simulink library "ox_lib"  (Simulink 7.5)
settings: Solver=ode45  SolverMode=SingleTasking  StartTime=0.0  StopTime=10.0  RelTol=1e-3
PostLoadFcn:
  | % Stub definitions for mask variables
  | delay_depth=16;
  | n_bits=8;
  | bin_pt=7;
libraries: xbsIndex_r4 x698, casper_library x173, ox_lib x8, xps_library x2
(part 1 of 8)
settings Model: Creator=mwagner  LastModifiedBy=jack

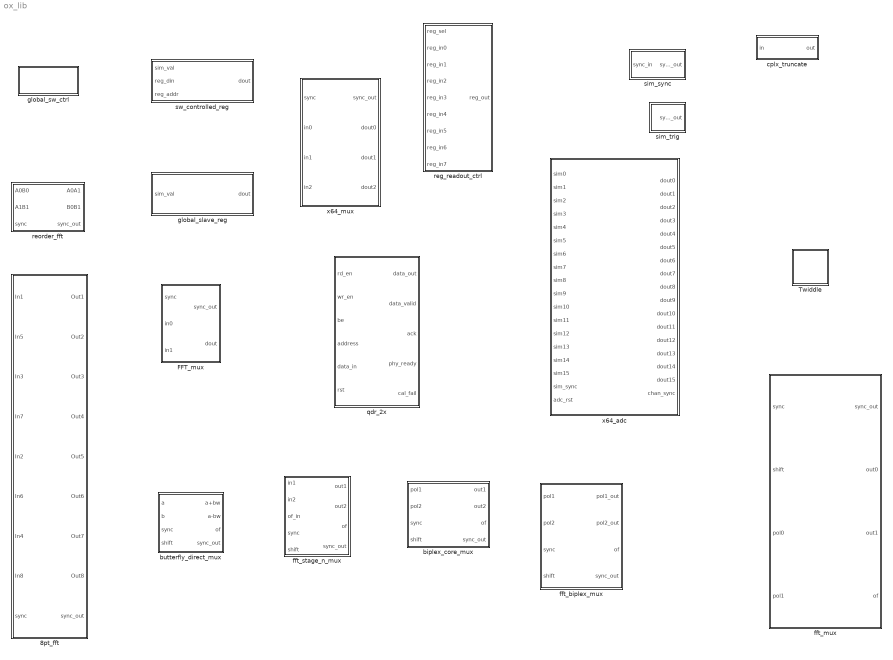
== system ox_lib ==
  8pt_fft : Subsystem
      mask Type: 8pt_fft
      mask Description:
      | Input 8 values and get 8 fourier components!
      | 
      | Simples!
      | 
      | [Latency 24]
  FFT_mux : Subsystem  mask{fft_len=9, fft_inputs=2, bit_width=18, bram_lat=2}
      mask prompts: fft_len "FFT length (2^?)"; fft_inputs "Number of FFT inputs (2^?) -- doesn't yet work for values other than 2"; bit_width "Bit width of samples"; bram_lat "bram latency"
  Twiddle : Subsystem
  biplex_core_mux : Subsystem  mask(biplex_core_mux){FFTSize=3, input_bit_width=18, coeff_bit_width=18, quantization=Truncate, overflow=Wrap, add_latency=1, mult_latency=2, bram_latency=3, arch=Virtex2Pro, opt_target=Multipliers, coeffs_bit_limit=8, delays_bit_limit=8, specify_mult=off, mult_spec=[2                                      2                                      2], dsp48_adders=off, mux_factor=0}
      mask prompts: FFTSize "Size of FFT: (2^? pnts)"; input_bit_width "Input/Output Bit Width"; coeff_bit_width "Coefficient Bit Width"; quantization "Quantization Behavior"; overflow "Overflow Behavior"; add_latency "Add Latency"; mult_latency "Mult Latency"; bram_latency "BRAM Latency"; arch "Architecture"; opt_target "Optimisation Target"; coeffs_bit_limit "Number bits above which to store stage's coefficients in BRAM (2^? bits)"; delays_bit_limit "Number bits above which to implent stage's delays in BRAM (2^? bits)"; specify_mult "Specify multiplier use (behavioural HDL if not specified)"; mult_spec "Multiplier specification (0=core, 1=embedded, 2=behavioural) (left=1st stage)"; dsp48_adders "Use DSP48s for adders"; mux_factor "Multiplex factor (2^?)"
      mask init:
      | biplex_core_mux_init(gcb,...
      |     'FFTSize', FFTSize,...
      |     'mux_factor', mux_factor, ...
      |     'input_bit_width', input_bit_width,...
      |     'coeff_bit_width', coeff_bit_width,...
      |     'quantization', quantization,...
      |     'overflow', overflow,...
      |     'add_latency', add_latency,...
      |     'mult_latency', mult_latency,...
      |     'bram_latency', bram_latency,...
      |     'arch', arch, ...
      |     'opt_target', opt_target, ...
      |     'coeffs_bit_limit', coeffs_bit_limit, ...
      |     'delays_bit_limit', delays_bit_limit, ...
      |     'specify_mult', specify_mult, ...
      |     'mult_spec', mult_spec, ...
      |     'dsp48_adders', dsp48_adders );
      settings: AttributesFormatString=|
      | FFTSize=3,
      |  opt_target=Multipliers,
      |  arch=Virtex2Pro
      mask StyleString: edit,edit,edit,popup(Truncate|Round  (unbiased: +/- Inf)|Round  (unbiased: Even Values)),popup(Wrap|Saturate|Error),edit,edit,edit,popup(Virtex2Pro|Virtex5),popup(Logic|Multipliers),edit,edit,checkbox,edit,checkbox,edit
      mask CallbackString:
      | % fft_size = eval(get_param(gcb, 'FFTSize'));
      | % old_vec = eval(get_param(gcb, 'mult_spec'));
      | 
      | % vec = 2.*ones(1,fft_size);
      | % old_size = length(old_vec);
      | 
      | % if(old_size <= fft_size),
      | %    size = old_size;
      | % else,
      | %     size = fft_size;
      | % end
      | 
      | % for n = 1:size, vec(n) = old_vec(n); end
      | % set_param(gcb, 'mult_spec', mat2str(vec));||||||||||||specify_mult = get_param(gcb,'specify_mult');
      | visibs = get_param(gcb,'MaskVisibilities');
      | if( strcmp(specify_mult,'off')), visibs{14} = 'off';
      | else, visibs{14} = 'on';
      | end
      | set_param(gcb, 'MaskVisibilities', visibs);
      | enables = get_param(gcb,'MaskVisibilities');
      | enables{14} = 'on';
      | set_param(gcb, 'MaskEnables', enables);
      | |% vec = eval( get_param(gcb, 'mult_spec'));
      | % vec_size = length(vec);
      | % fft_size = eval( get_param(gcb, 'FFTSize'));
      | % new_vec = 2.*ones(1, fft_size);
      | 
      | % if(vec_size <= fft_size), size = vec_size;
      | % else size = fft_size;
      | % end
      | 
      | % for n=1:size
      | %     new_vec(n) = vec(n);
      | % end
      | % set_param(gcb, 'mult_spec', mat2str(new_vec));||
  butterfly_direct_mux : Subsystem  mask(butterfly_direct_mux){biplex=on, FFTSize=4, Coeffs=0, coeff_bit_width=18, StepPeriod=3, bram_latency=3, coeffs_bram=off, input_bit_width=18, add_latency=1, mult_latency=3, quantization=Truncate, overflow=Wrap, arch=Virtex2Pro, opt_target=Multipliers, use_hdl=on, use_embedded=off, dsp48_adders=off, mux_factor=0}
      mask prompts: biplex "Used in biplex FFT"; FFTSize "Size of FFT: (2^?)"; Coeffs "Coefficients: (0 to 2^(FFTSize-1)-1)"; coeff_bit_width "Coefficient Bit Width"; StepPeriod "Coefficient Step Period: (2^?)"; bram_latency "BRAM Latency"; coeffs_bram "Implement coefficients in BRAM"; input_bit_width "Input/Output Bit Width:"; add_latency "Add Latency"; mult_latency "Mult Latency"; quantization "Quantization Behavior"; overflow "Overflow Behavior"; arch "Architecture"; opt_target "Optimisation target"; use_hdl "Use behavioural HDL for multipliers"; use_embedded "Use embedded multipliers"; dsp48_adders "Use DSP48s for adders"; mux_factor "Multiplex factor (2^?)"
      mask init:
      | butterfly_direct_mux_init(gcb,...
      |               'biplex', biplex,...
      |               'FFTSize', FFTSize,...
      |               'mux_factor', mux_factor, ...
      |               'Coeffs', Coeffs,...
      |               'coeff_bit_width', coeff_bit_width,...
      |               'StepPeriod', StepPeriod,...
      |               'bram_latency', bram_latency,...
      |               'coeffs_bram', coeffs_bram,...
      |               'input_bit_width', input_bit_width,...
      |               'add_latency', add_latency,...
      |               'mult_latency', mult_latency,...
      |               'quantization', quantization,...
      |               'overflow', overflow,...
      |               'arch', arch,...
      |               'opt_target', opt_target,...
      |               'use_hdl', use_hdl,...
      |               'use_embedded', use_embedded,...
      |               'dsp48_adders', dsp48_adders);
      settings: AttributesFormatString=FFTSize=4, coeff_bit_width=18
      mask StyleString: checkbox,edit,edit,edit,edit,edit,checkbox,edit,edit,edit,popup(Truncate|Round  (unbiased: +/- Inf)|Round  (unbiased: Even Values)),popup(Wrap|Saturate|Error),popup(Virtex2Pro|Virtex5),popup(Logic|Multipliers),checkbox,checkbox,checkbox,edit
      mask CallbackString:
      | ||coeffs = eval(get_param(gcb,'Coeffs'));
      | visibs = get_param(gcb,'MaskVisibilities');
      | if length(coeffs) == 1,
      |     visibs{5} = 'off'; visibs{6} = 'off';
      |     visibs{7} = 'off';
      | else
      |     visibs{5} = 'on';
      |     visibs{6} = 'on'; visibs{7} = 'on';
      | end
      | set_param(gcb, 'MaskVisibilities', visibs);||||||||||||use_hdl = get_param(gcb,'use_hdl');
      | visibs = get_param(gcb, 'MaskVisibilities');
      | if( strcmp(use_hdl,'on')),
      |     set_param(gcb, 'use_embedded','off');
      |     visibs{16} = 'off';
      | else,
      |     visibs{16} = 'on';
      | end
      |     set_param(gcb, 'MaskVisibilities',visibs);|||
  cplx_truncate : Subsystem  mask{in_bits=19, out_bits=16}
      mask prompts: in_bits "Input bitwidth"; out_bits "Output bitwidth"
  fft_biplex_mux : Subsystem  mask(fft_biplex_mux){FFTSize=4, mux_factor=2, input_bit_width=18, coeff_bit_width=18, quantization=Truncate, overflow=Wrap, add_latency=1, mult_latency=3, bram_latency=3, arch=Virtex2Pro, opt_target=Multipliers, coeffs_bit_limit=8, delays_bit_limit=9, specify_mult=off, mult_spec=getfield( getfield( get_param( gcb,'UserData' ), 'parameters'),'mult_spec'), dsp48_adders=off}
      mask prompts: FFTSize "Size of FFT: (2^? pnts)"; mux_factor "Multiplexing factor (2^?)"; input_bit_width "Input/Output Bit Width"; coeff_bit_width "Coefficient Bit Width"; quantization "Quantization Behavior"; overflow "Overflow Behavior"; add_latency "Add Latency"; mult_latency "Mult Latency"; bram_latency "BRAM Latency"; arch "Architecture"; opt_target "Optimisation Target"; coeffs_bit_limit "Number bits above which to store stage's coefficients in BRAM (2^? bits)"; delays_bit_limit "Number bits above which to implent stage's delays in BRAM (2^? bits)"; specify_mult "Specify multiplier use (behavioral HDL if not specified)"; mult_spec "Multiplier specification (0=core, 1=embedded, 2=behavioural) (left=1st stage)"; dsp48_adders "Use DSP48s for adders"
      mask init:
      | fft_biplex_mux_init(gcb,...
      |     'FFTSize', FFTSize,...
      |     'mux_factor', mux_factor,...
      |     'input_bit_width', input_bit_width,...
      |     'coeff_bit_width', coeff_bit_width,...
      |     'quantization', quantization,...
      |     'overflow', overflow,...
      |     'add_latency', add_latency,...
      |     'mult_latency', mult_latency,...
      |     'bram_latency', bram_latency,...
      |     'arch', arch, ...
      |     'opt_target', opt_target, ...
      |     'coeffs_bit_limit', coeffs_bit_limit, ...
      |     'delays_bit_limit', delays_bit_limit, ...
      |     'specify_mult', specify_mult,...
      |     'mult_spec', mult_spec, ...
      |     'dsp48_adders', dsp48_adders);
      settings: AttributesFormatString=|
      | FFTSize=4,
      |  arch=Virtex2Pro,
      |  opt_target=Multipliers
      mask StyleString: edit,edit,edit,edit,popup(Truncate|Round  (unbiased: +/- Inf)|Round  (unbiased: Even Values)),popup(Wrap|Saturate|Error),edit,edit,edit,popup(Virtex2Pro|Virtex5),popup(Logic|Multipliers),edit,edit,checkbox,edit,checkbox
      mask CallbackString:
      | % fft_size = eval(get_param(gcb, 'FFTSize'));
      | % old_vec = eval(get_param(gcb, 'mult_spec'));
      | 
      | % vec = 2.*ones(1,fft_size);
      | % old_size = length(old_vec);
      | 
      | % if(old_size <= fft_size),
      | %    size = old_size;
      | % else,
      | %     size = fft_size;
      | % end
      | 
      | % for n = 1:size, vec(n) = old_vec(n); end
      | % set_param(gcb, 'mult_spec', mat2str(vec));|||||||||||||specify_mult = get_param(gcb,'specify_mult');
      | visibs = get_param(gcb, 'MaskVisibilities');
      | 
      | if( strcmp(specify_mult,'off')), visibs{14} = 'off';
      | else, visibs{14} = 'on';
      | end
      | set_param(gcb, 'MaskVisibilities', visibs);
      | |% vec = eval( get_param(gcb, 'mult_spec'));
      | % vec_size = length(vec);
      | % fft_size = eval( get_param(gcb, 'FFTSize'));
      | % new_vec = 2.*ones(1, fft_size);
      | 
      | % if(vec_size <= fft_size), size = vec_size;
      | % else size = fft_size;
      | % end
      | 
      | % for n=1:size
      | %     new_vec(n) = vec(n);
      | % end
      | % set_param(gcb, 'mult_spec', mat2str(new_vec));|
  fft_mux : Subsystem  mask(fft_mux){FFTSize=4, mux_factor=0, input_bit_width=18, coeff_bit_width=18, n_inputs=0, quantization=Truncate, overflow=Wrap, add_latency=1, mult_latency=3, bram_latency=3, arch=Virtex2Pro, opt_target=Multipliers, coeffs_bit_limit=8, delays_bit_limit=9, specify_mult=off, mult_spec=[2                                      2                                      2], dsp48_adders=off}
      mask prompts: FFTSize "Size of FFT: (2^?)"; mux_factor "Multiplex factor (2^?)"; input_bit_width "Input/Output Bit Width"; coeff_bit_width "Coefficient Bit Width"; n_inputs "Number of Simultaneous Inputs: (2^?)"; quantization "Quantization Behavior"; overflow "Overflow Behavior"; add_latency "Add Latency"; mult_latency "Mult Latency"; bram_latency "BRAM Latency"; arch "Architecture"; opt_target "Optimisation Target"; coeffs_bit_limit "Number bits above which to store stage's coefficients in BRAM (2^? bits)"; delays_bit_limit "Number bits above which to store stage's delays in BRAM (2^? bits)"; specify_mult "Specify multiplier use (behavioral HDL if not specified)"; mult_spec "Multiplier specification (0=core, 1=embedded, 2=behavioural) (left=1st stage)"; dsp48_adders "Use DSP48s for adders"
      mask init:
      | fft_mux_init(gcb,...
      |     'FFTSize', FFTSize, ...
      |     'mux_factor', mux_factor,...
      |     'input_bit_width', input_bit_width, ...
      |     'coeff_bit_width', coeff_bit_width, ...
      |     'n_inputs', n_inputs, ...
      |     'quantization', quantization, ...
      |     'overflow', overflow, ...
      |     'add_latency', add_latency, ...
      |     'mult_latency', mult_latency, ...
      |     'bram_latency', bram_latency, ...
      |     'arch', arch, ...
      |     'opt_target', opt_target, ...
      |     'coeffs_bit_limit', coeffs_bit_limit, ...
      |     'delays_bit_limit', delays_bit_limit, ...
      |     'specify_mult', specify_mult, ...
      |     'mult_spec', mult_spec, ...
      |     'dsp48_adders', dsp48_adders);
      settings: AttributesFormatString=FFTSize=4, n_inputs=0
      mask Help: eval('xlWeb(''http://casper.berkeley.edu/wiki/Fft'')')
      mask StyleString: edit,edit,edit,edit,edit,popup(Truncate|Round  (unbiased: +/- Inf)|Round  (unbiased: Even Values)),popup(Wrap|Saturate|Error),edit,edit,edit,popup(Virtex2Pro|Virtex5),popup(Logic|Multipliers),edit,edit,checkbox,edit,checkbox
      mask CallbackString:
      | % fft_size = eval(get_param(gcb, 'FFTSize'));
      | % old_vec = eval(get_param(gcb, 'mult_spec'));
      | 
      | % vec = 2.*ones(1,fft_size);
      | % old_size = length(old_vec);
      | 
      | % if(old_size <= fft_size), size = old_size;
      | % else, size = fft_size;
      | % end
      | 
      | % for n = 1:size, vec(n) = old_vec(n); end
      | % set_param(gcb, 'mult_spec', mat2str(vec));||||||||||||||specify_mult = get_param(gcb,'specify_mult');
      | visibs = get_param(gcb, 'MaskVisibilities');
      | if( strcmp(specify_mult,'off')), visibs{15} = 'off';
      | else visibs{15} = 'on';
      | end
      | set_param(gcb, 'MaskVisibilities', visibs);
      | 
      | |% vec = eval( get_param(gcb, 'mult_spec'));
      | % vec_size = length(vec);
      | % fft_size = eval( get_param(gcb, 'FFTSize'));
      | % new_vec = 2.*ones(1, fft_size);
      | 
      | % if(vec_size <= fft_size), size = vec_size;
      | % else size = fft_size;
      | % end
      | 
      | % for n=1:size,
      | %    new_vec(n) = vec(n);
      | % end
      | % set_param(gcb, 'mult_spec', mat2str(new_vec));|
  fft_stage_n_mux : Subsystem  mask(fft_stage_n_mux){FFTSize=4, FFTStage=1, input_bit_width=18, coeff_bit_width=18, delays_bram=off, coeffs_bram=off, MaxCoeffNum=16, quantization=Truncate, overflow=Wrap, add_latency=1, mult_latency=3, bram_latency=3, arch=Virtex2Pro, opt_target=Multipliers, use_hdl=on, use_embedded=off, dsp48_adders=off, mux_factor=4}
      mask prompts: FFTSize "Size of FFT: (2^? pnts)"; FFTStage "Stage of FFT:"; input_bit_width "Input/Output Bit Width:"; coeff_bit_width "Coefficient Bit Width"; delays_bram "Implement Delays in BRAM:"; coeffs_bram "Store Coefficients in BRAM:"; MaxCoeffNum "Maximum Coefficient Depth: (2^?)"; quantization "Quantization Behavior"; overflow "Overflow Behavior"; add_latency "Add Latency"; mult_latency "Mult Latency"; bram_latency "BRAM Latency"; arch "Architecture"; opt_target "Optimisation target"; use_hdl "Use behavioural HDL for mutlipliers"; use_embedded "Use embedded multipliers"; dsp48_adders "Use DSP48s for adders"; mux_factor "Multiplex factor (2^?)"
      mask init:
      | fft_stage_n_mux_init(gcb,...
      |     'FFTSize', FFTSize,...
      |     'mux_factor', mux_factor, ...
      |     'FFTStage', FFTStage,...
      |     'input_bit_width', input_bit_width,...
      |     'coeff_bit_width', coeff_bit_width,...
      |     'delays_bram', delays_bram,...
      |     'coeffs_bram', coeffs_bram,...
      |     'MaxCoeffNum', MaxCoeffNum,...
      |     'quantization', quantization,...
      |     'overflow', overflow,...
      |     'add_latency', add_latency,...
      |     'mult_latency', mult_latency,...
      |     'bram_latency', bram_latency,...
      |     'arch', arch, ...
      |     'opt_target', opt_target, ...
      |     'use_hdl', use_hdl,...
      |     'use_embedded', use_embedded, ...
      |     'dsp48_adders', dsp48_adders);
      settings: AttributesFormatString=|
      | FFTSize=4, FFTStage=1,
      |  coeffs_bram=off,
      |  delays_bram=off
      mask StyleString: edit,edit,edit,edit,checkbox,checkbox,edit,popup(Truncate|Round  (unbiased: +/- Inf)|Round  (unbiased: Even Values)),popup(Wrap|Saturate|Error),edit,edit,edit,popup(Virtex2Pro|Virtex5),popup(Logic|Multipliers),checkbox,checkbox,checkbox,edit
      mask CallbackString:
      | ||||||||||||||use_hdl = get_param(gcb,'use_hdl');
      | visibs = get_param(gcb, 'MaskVisibilities');
      | if( strcmp(use_hdl,'on')),
      |     visibs{16} = 'off';
      | else,
      |     visibs{16} = 'on';
      | end
      |     set_param(gcb, 'MaskVisibilities',visibs);|||
  global_slave_reg : Subsystem  mask{reg_name=My Register, data_width=32, latency=0, auto=off, enable_bit=0}
      mask prompts: reg_name "Register Name"; data_width "Data width (bits): 1-32"; latency "Pipelined delay (0 for none)"; auto "Use automatic addressing? (not yet implemented)"; enable_bit "Address Number: 0-31"
      mask init:
      | pipeline_init([gcb '/pipeline1'], 'latency', latency);
      | pipeline_init([gcb '/pipeline2'], 'latency', latency);
      | 
      | fmtstr = sprintf('Name: %s, Number :%d, Latency:%d', reg_name, enable_bit, latency);
      | 
      | set_param(gcb, 'AttributesFormatString', fmtstr);
      settings: AttributesFormatString=Name: My Register, Number :0, Latency:10
  global_sw_ctrl : Subsystem
      settings: PermitHierarchicalResolution=None
      mask Type: global_sw_reg
      mask Description: The beginnings of a lightweight control system for designs with many software registers.
  qdr_2x : Subsystem  Tag=xps:qdr_2x  mask(qdr_2x){which_qdr=qdr0, qdr_awidth=12, use_sniffer=off}
      mask prompts: which_qdr "QDR Chip"; qdr_awidth "Simulation QDR address width"; use_sniffer "Include CPU Interface"
      mask help: Interface to the QDR II SRAM device on ROACH, with 2x multiplexing
      mask init:
      | qdr_2x_mask(gcb);
      mask StyleString: popup(qdr0|qdr1),edit,checkbox
  reg_readout_ctrl : Subsystem  mask{n_registers=8, mux_latency=2}
      mask prompts: n_registers "Number of register inputs"; mux_latency "mux latency"
      mask init:
      | reg_readout_ctrl_init(gcb, ...
      |     'n_registers', n_registers, ...
      |     'mux_latency', mux_latency);
      settings: AttributesFormatString=|
      | n_inputs=8
      | latency=2
  reorder_fft : Subsystem  mask{N=256}
      mask prompts: N "window size"
  sim_sync : Subsystem  mask{delay=1}
      mask prompts: delay "time of pulse (clocks from simulation start)"
  sim_trig : Subsystem  mask{delay=1}
      mask prompts: delay "time of pulse (clocks from simulation start)"
  sw_controlled_reg : Subsystem  mask{reg_name=My Register, enable_bit=0, data_width=32}
      mask prompts: reg_name "Register Name"; enable_bit "Address Number: 0-31"; data_width "Data width (bits): 1-32"
      mask init:
      | fmtstr = sprintf('Name: %s\nNumber :%d', reg_name, enable_bit);
      | 
      | set_param(gcb, 'AttributesFormatString', fmtstr);
      settings: AttributesFormatString=|
      | Name: My Register
      | Number :0
  x64_adc : Subsystem  Tag=xps:x64_adc  mask(x64_adc){adc_clk_rate=64, spi=off, ctrl_gpio=GPIO_A}
      mask prompts: adc_clk_rate "ADC clock rate (MHz)"; spi "Include SPI interface?"; ctrl_gpio "GPIO bank to use for control signals?"
      mask help: The ADC block converts analog inputs to digital outputs. Every clock cycle, the inputs are sampled and digitized to 8 bit binary point numbers in the range of [-1, 1) and are then output by the adc.
      mask init:
      | x64_adc_mask(gcb);
      mask Help: eval('xlWeb([getenv(''MLIB_ROOT''), ''\doc\html\sys_adc\sys_adc.html''])')
      mask StyleString: edit,checkbox,popup(GPIO_A|GPIO_B)
  x64_mux : Subsystem  mask{fft_len=2, bram_lat=2}
      mask prompts: fft_len "FFT length (2^?)"; bram_lat "bram latency"

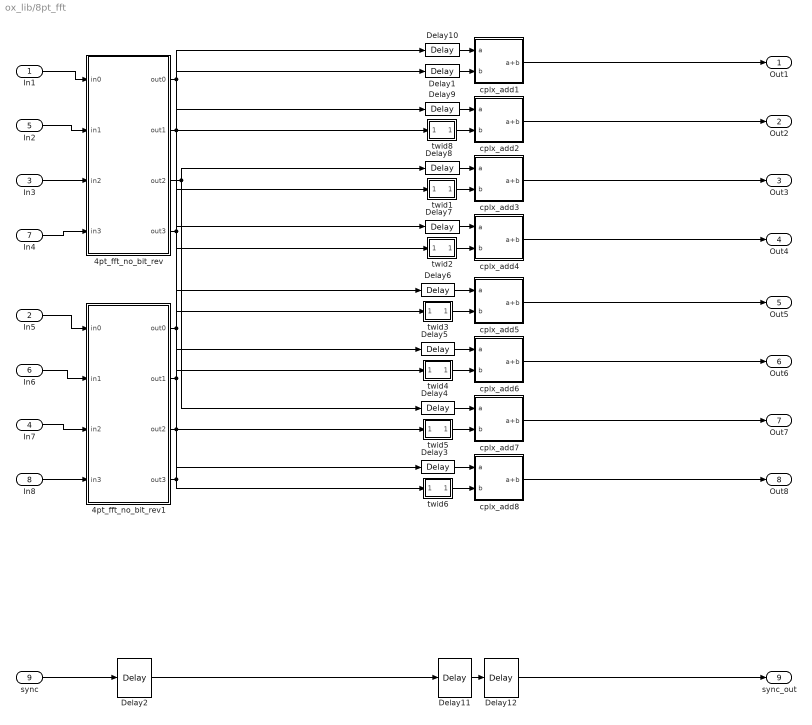
== system ox_lib/8pt_fft ==
  In1 : Inport  OutDataType=sfix(16)  OutScaling=2^0
  In5 : Inport  Port=2  OutDataType=sfix(16)  OutScaling=2^0
  In3 : Inport  Port=3  OutDataType=sfix(16)  OutScaling=2^0
  In7 : Inport  Port=4  OutDataType=sfix(16)  OutScaling=2^0
  In2 : Inport  Port=5  OutDataType=sfix(16)  OutScaling=2^0
  In6 : Inport  Port=6  OutDataType=sfix(16)  OutScaling=2^0
  In4 : Inport  Port=7  OutDataType=sfix(16)  OutScaling=2^0
  In8 : Inport  Port=8  OutDataType=sfix(16)  OutScaling=2^0
  sync : Inport  Port=9  OutDataType=sfix(16)  OutScaling=2^0
  4pt_fft_no_bit_rev : Subsystem
  4pt_fft_no_bit_rev1 : Subsystem
  Delay{1,3..11} (10 alike) : xbsIndex_r4/Delay  en=off  latency=8  dbl_ovrd=off  reg_retiming=off  block_type=delay
      settings: block_version=11.4
  Delay12 : xbsIndex_r4/Delay  en=off  latency=4  dbl_ovrd=off  reg_retiming=off  block_type=delay
      settings: block_version=11.4
  Delay2 : xbsIndex_r4/Delay  en=off  latency=12  dbl_ovrd=off  reg_retiming=off  block_type=delay
      settings: block_version=11.4
  cplx_add1 : Subsystem  AncestorBlock=casper_library/Misc/complex_addsub  mask(cplx_add){BitWidth=8, add_latency=2}
      mask prompts: BitWidth "Bit Wdith"; add_latency "Add Latency"
  cplx_add2 : Subsystem  AncestorBlock=casper_library/Misc/complex_addsub  mask(cplx_add){BitWidth=8, add_latency=2}
      mask prompts: BitWidth "Bit Wdith"; add_latency "Add Latency"
  cplx_add3 : Subsystem  AncestorBlock=casper_library/Misc/complex_addsub  mask(cplx_add){BitWidth=8, add_latency=2}
      mask prompts: BitWidth "Bit Wdith"; add_latency "Add Latency"
  cplx_add4 : Subsystem  AncestorBlock=casper_library/Misc/complex_addsub  mask(cplx_add){BitWidth=8, add_latency=2}
      mask prompts: BitWidth "Bit Wdith"; add_latency "Add Latency"
  cplx_add5 : Subsystem  AncestorBlock=casper_library/Misc/complex_addsub  mask(cplx_add){BitWidth=8, add_latency=2}
      mask prompts: BitWidth "Bit Wdith"; add_latency "Add Latency"
  cplx_add6 : Subsystem  AncestorBlock=casper_library/Misc/complex_addsub  mask(cplx_add){BitWidth=8, add_latency=2}
      mask prompts: BitWidth "Bit Wdith"; add_latency "Add Latency"
  cplx_add7 : Subsystem  AncestorBlock=casper_library/Misc/complex_addsub  mask(cplx_add){BitWidth=8, add_latency=2}
      mask prompts: BitWidth "Bit Wdith"; add_latency "Add Latency"
  cplx_add8 : Subsystem  AncestorBlock=casper_library/Misc/complex_addsub  mask(cplx_add){BitWidth=8, add_latency=2}
      mask prompts: BitWidth "Bit Wdith"; add_latency "Add Latency"
  twid1 : Subsystem  mask{phase=-2*pi/4}
      mask init:
      | fmtstr = sprintf('twiddle_phase: %d', phase);
      | set_param(gcb, 'AttributesFormatString', fmtstr);
      settings: AttributesFormatString=twiddle_phase: -1.570796e+00
  twid2 : Subsystem  mask{phase=-3*pi/4}
      mask init:
      | fmtstr = sprintf('twiddle_phase: %d', phase);
      | set_param(gcb, 'AttributesFormatString', fmtstr);
      settings: AttributesFormatString=twiddle_phase: -2.356194e+00
  twid3 : Subsystem  mask{phase=-4*pi/4}
      mask init:
      | fmtstr = sprintf('twiddle_phase: %d', phase);
      | set_param(gcb, 'AttributesFormatString', fmtstr);
      settings: AttributesFormatString=twiddle_phase: -3.141593e+00
  twid4 : Subsystem  mask{phase=-5*pi/4}
      mask init:
      | fmtstr = sprintf('twiddle_phase: %d', phase);
      | set_param(gcb, 'AttributesFormatString', fmtstr);
      settings: AttributesFormatString=twiddle_phase: -3.926991e+00
  twid5 : Subsystem  mask{phase=-6*pi/4}
      mask init:
      | fmtstr = sprintf('twiddle_phase: %d', phase);
      | set_param(gcb, 'AttributesFormatString', fmtstr);
      settings: AttributesFormatString=twiddle_phase: -4.712389e+00
  twid6 : Subsystem  mask{phase=-7*pi/4}
      mask init:
      | fmtstr = sprintf('twiddle_phase: %d', phase);
      | set_param(gcb, 'AttributesFormatString', fmtstr);
      settings: AttributesFormatString=twiddle_phase: -5.497787e+00
  twid8 : Subsystem  mask{phase=-pi/4}
      mask init:
      | fmtstr = sprintf('twiddle_phase: %d', phase);
      | set_param(gcb, 'AttributesFormatString', fmtstr);
      settings: AttributesFormatString=twiddle_phase: -7.853982e-01
  Out1 : Outport  OutDataType=sfix(16)  OutScaling=2^0
  Out2 : Outport  Port=2  OutDataType=sfix(16)  OutScaling=2^0
  Out3 : Outport  Port=3  OutDataType=sfix(16)  OutScaling=2^0
  Out4 : Outport  Port=4  OutDataType=sfix(16)  OutScaling=2^0
  Out5 : Outport  Port=5  OutDataType=sfix(16)  OutScaling=2^0
  Out6 : Outport  Port=6  OutDataType=sfix(16)  OutScaling=2^0
  Out7 : Outport  Port=7  OutDataType=sfix(16)  OutScaling=2^0
  Out8 : Outport  Port=8  OutDataType=sfix(16)  OutScaling=2^0
  sync_out : Outport  Port=9  OutDataType=sfix(16)  OutScaling=2^0
  wires:
  Delay10/1 -> cplx_add1/1(a)
  Delay9/1 -> cplx_add2/1(a)
  Delay8/1 -> cplx_add3/1(a)
  Delay7/1 -> cplx_add4/1(a)
  Delay6/1 -> cplx_add5/1(a)
  Delay5/1 -> cplx_add6/1(a)
  Delay4/1 -> cplx_add7/1(a)
  Delay3/1 -> cplx_add8/1(a)
  cplx_add8/1(a+b) -> Out8/1
  cplx_add7/1(a+b) -> Out7/1
  cplx_add6/1(a+b) -> Out6/1
  cplx_add5/1(a+b) -> Out5/1
  cplx_add4/1(a+b) -> Out4/1
  cplx_add3/1(a+b) -> Out3/1
  cplx_add2/1(a+b) -> Out2/1
  cplx_add1/1(a+b) -> Out1/1
  twid6/1(Out1) -> cplx_add8/2(b)
  twid5/1(Out1) -> cplx_add7/2(b)
  twid4/1(Out1) -> cplx_add6/2(b)
  twid3/1(Out1) -> cplx_add5/2(b)
  twid2/1(Out1) -> cplx_add4/2(b)
  twid1/1(Out1) -> cplx_add3/2(b)
  twid8/1(Out1) -> cplx_add2/2(b)
  Delay1/1 -> cplx_add1/2(b)
  sync/1 -> Delay2/1
  Delay2/1 -> Delay11/1
  Delay11/1 -> Delay12/1
  Delay12/1 -> sync_out/1
  In1/1 -> 4pt_fft_no_bit_rev/1(in0)
  In5/1 -> 4pt_fft_no_bit_rev1/1(in0)
  In6/1 -> 4pt_fft_no_bit_rev1/2(in1)
  In7/1 -> 4pt_fft_no_bit_rev1/3(in2)
  In8/1 -> 4pt_fft_no_bit_rev1/4(in3)
  4pt_fft_no_bit_rev/1(out0) -> Delay10/1, Delay6/1
  4pt_fft_no_bit_rev/2(out1) -> Delay9/1, Delay5/1
  4pt_fft_no_bit_rev/3(out2) -> Delay8/1, Delay4/1
  4pt_fft_no_bit_rev/4(out3) -> Delay7/1, Delay3/1
  4pt_fft_no_bit_rev1/1(out0) -> twid3/1(In1), Delay1/1
  4pt_fft_no_bit_rev1/2(out1) -> twid4/1(In1), twid8/1(In1)
  4pt_fft_no_bit_rev1/3(out2) -> twid5/1(In1), twid1/1(In1)
  4pt_fft_no_bit_rev1/4(out3) -> twid6/1(In1), twid2/1(In1)
  In2/1 -> 4pt_fft_no_bit_rev/2(in1)
  In3/1 -> 4pt_fft_no_bit_rev/3(in2)
  In4/1 -> 4pt_fft_no_bit_rev/4(in3)

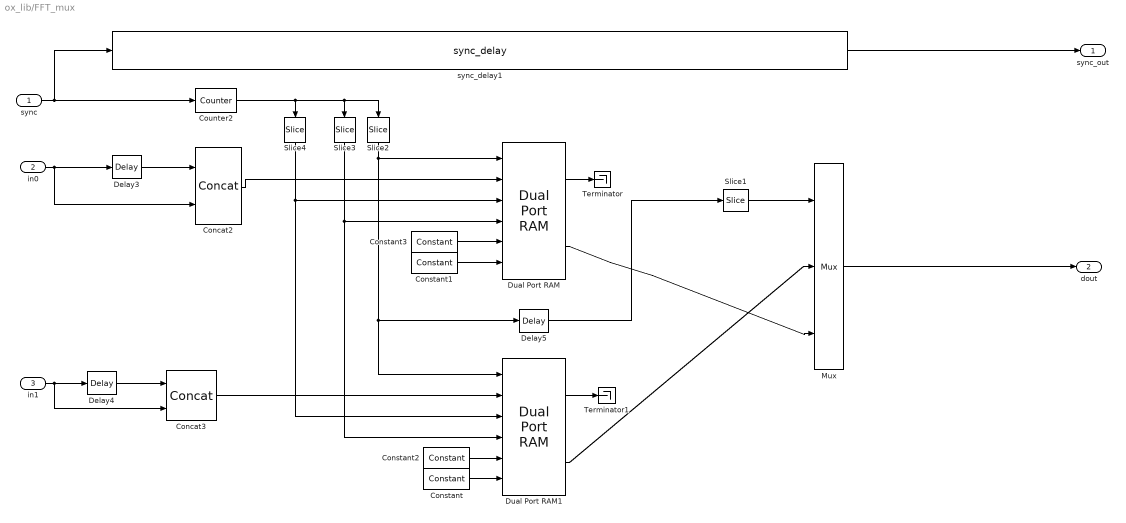
== system ox_lib/FFT_mux ==
  sync : Inport  OutDataType=fixdt(1, 16)  OutScaling=2^0
  in0 : Inport  Port=2  OutDataType=fixdt(1, 16)  OutScaling=2^0
  in1 : Inport  Port=3  OutDataType=fixdt(1, 16)  OutScaling=2^0
  Concat2 : xbsIndex_r4/Concat  num_inputs=2  dbl_ovrd=off  block_type=concat
  Concat3 : xbsIndex_r4/Concat  num_inputs=2  dbl_ovrd=off  block_type=concat
  Constant : xbsIndex_r4/Constant  arith_type=Boolean  const=0  n_bits=16  bin_pt=14  explicit_period=off  period=1  equ=P=C  opselect=C  inp2=PCIN>>17  opr=+  inp1=P  carry=CIN  dbl_ovrd=off  block_type=constant
      settings: block_version=11.4
  Constant1 : xbsIndex_r4/Constant  arith_type=Boolean  const=0  n_bits=16  bin_pt=14  explicit_period=off  period=1  equ=P=C  opselect=C  inp2=PCIN>>17  opr=+  inp1=P  carry=CIN  dbl_ovrd=off  block_type=constant
      settings: block_version=11.4
  Constant2 : xbsIndex_r4/Constant  arith_type=Unsigned  const=0  n_bits=(2^fft_inputs)*bit_width  bin_pt=0  explicit_period=on  period=1  equ=P=C  opselect=C  inp2=PCIN>>17  opr=+  inp1=P  carry=CIN  dbl_ovrd=off  block_type=constant
      settings: block_version=11.4
  Constant3 : xbsIndex_r4/Constant  arith_type=Unsigned  const=0  n_bits=(2^fft_inputs)*bit_width  bin_pt=0  explicit_period=on  period=1  equ=P=C  opselect=C  inp2=PCIN>>17  opr=+  inp1=P  carry=CIN  dbl_ovrd=off  block_type=constant
      settings: block_version=11.4
  Counter2 : xbsIndex_r4/Counter  cnt_type=Free Running  cnt_to=Inf  operation=Up  start_count=0  cnt_by_val=1  arith_type=Unsigned  n_bits=fft_len-fft_inputs+1  bin_pt=0  load_pin=off  rst=on  en=off  explicit_period=on  period=1  dbl_ovrd=off  use_behavioral_HDL=off  implementation=Fabric  block_type=counter
      settings: block_version=11.4
  Delay3 : xbsIndex_r4/Delay  en=off  latency=1  dbl_ovrd=off  reg_retiming=off  block_type=delay
      settings: block_version=11.4
  Delay4 : xbsIndex_r4/Delay  en=off  latency=1  dbl_ovrd=off  reg_retiming=off  block_type=delay
      settings: block_version=11.4
  Delay5 : xbsIndex_r4/Delay  en=off  latency=bram_lat  dbl_ovrd=off  reg_retiming=off  block_type=delay
      settings: block_version=11.4
  Dual Port RAM : xbsIndex_r4/Dual Port RAM  depth=2^(fft_len-fft_inputs)  initVector=0  distributed_mem=Block RAM  init_a=0  init_b=0  rst_a=off  rst_b=off  en_a=off  en_b=off  latency=bram_lat  write_mode_A=Read Before Write  write_mode_B=Read Before Write  dbl_ovrd=off  optimize=Area  use_rpm=on  block_type=dpram
      settings: block_version=11.4
  Dual Port RAM1 : xbsIndex_r4/Dual Port RAM  depth=2^(fft_len-fft_inputs)  initVector=0  distributed_mem=Block RAM  init_a=0  init_b=0  rst_a=off  rst_b=off  en_a=off  en_b=off  latency=bram_lat  write_mode_A=Read Before Write  write_mode_B=Read Before Write  dbl_ovrd=off  optimize=Area  use_rpm=on  block_type=dpram
      settings: block_version=11.4
  Mux : xbsIndex_r4/Mux  inputs=2  en=off  latency=1  precision=Full  arith_type=Unsigned  n_bits=16  bin_pt=14  quantization=Truncate  overflow=Wrap  dbl_ovrd=off  block_type=mux
      settings: block_version=11.4
  Slice1 : xbsIndex_r4/Slice  nbits=1  boolean_output=off  mode=Upper Bit Location + Width  bit1=0  base1=MSB of Input  bit0=0  base0=LSB of Input  dbl_ovrd=off  block_type=slice
  Slice2 : xbsIndex_r4/Slice  nbits=fft_len-fft_inputs  boolean_output=off  mode=Upper Bit Location + Width  bit1=0  base1=MSB of Input  bit0=0  base0=LSB of Input  dbl_ovrd=off  block_type=slice
  Slice3 : xbsIndex_r4/Slice  nbits=fft_len-fft_inputs  boolean_output=off  mode=Lower Bit Location + Width  bit1=0  base1=MSB of Input  bit0=0  base0=LSB of Input  dbl_ovrd=off  block_type=slice
  Slice4 : xbsIndex_r4/Slice  nbits=1  boolean_output=on  mode=Lower Bit Location + Width  bit1=0  base1=MSB of Input  bit0=0  base0=LSB of Input  dbl_ovrd=off  block_type=slice
  Terminator : Terminator
  Terminator1 : Terminator
  sync_delay1 : casper_library/Delays/sync_delay  SystemSampleTime=-1  DelayLen=2^(fft_len-fft_inputs)+bram_lat+1
  sync_out : Outport
  dout : Outport  Port=2
  wires:
  Dual Port RAM1/1 -> Terminator1/1
  Dual Port RAM/1 -> Terminator/1
  Delay5/1 -> Slice1/1
  sync_delay1/1 -> sync_out/1
  Mux/1 -> dout/1
  Slice1/1 -> Mux/1
  Constant3/1 -> Dual Port RAM/5
  Constant2/1 -> Dual Port RAM1/5
  Constant1/1 -> Dual Port RAM/6
  Constant/1 -> Dual Port RAM1/6
  Slice4/1 -> Dual Port RAM1/3, Dual Port RAM/3
  Slice3/1 -> Dual Port RAM1/4, Dual Port RAM/4
  Slice2/1 -> Delay5/1, Dual Port RAM1/1, Dual Port RAM/1
  Counter2/1 -> Slice4/1, Slice3/1, Slice2/1
  sync/1 -> sync_delay1/1, Counter2/1
  Concat3/1 -> Dual Port RAM1/2
  in1/1 -> Delay4/1, Concat3/2
  Delay4/1 -> Concat3/1
  Concat2/1 -> Dual Port RAM/2
  in0/1 -> Delay3/1, Concat2/2
  Delay3/1 -> Concat2/1
  Dual Port RAM/2 -> Mux/3
  Dual Port RAM1/2 -> Mux/2

== system ox_lib/Twiddle ==
  coeff_gen : Subsystem
  twiddle_coeff_0 : Subsystem  mask(twiddle_coeff_0){input_bit_width=18, coeff_bit_width=, add_latency=3, mult_latency=4, bram_latency=4, use_hdl=off, use_embedded=off, quantization=Truncate, overflow=Wrap, mux_factor=0}
      mask prompts: input_bit_width "Input Bit Width"; coeff_bit_width "Coefficient Bit Width"; add_latency "Add Latency"; mult_latency "Mult Latency"; bram_latency "BRAM Latency"; use_hdl "Use behavioural HDL for multipliers"; use_embedded "Use embedded multipliers"; quantization "Quantization Behavior"; overflow "Overflow Behavior"; mux_factor "Multiplex factor (2^?)"
      mask help:
      | Used in FFT library. Used when coefficients
      | are 2^0 i.e just pass data through
      mask StyleString: edit,edit,edit,edit,edit,checkbox,checkbox,popup(Truncate|Round  (unbiased: +/- Inf)|Round  (unbiased: Even Values)),popup(Wrap|Saturate|Error),edit
  twiddle_coeff_1 : Subsystem  mask(twiddle_coeff_1){input_bit_width=18, coeff_bit_width=, add_latency=3, mult_latency=4, bram_latency=4, use_hdl=off, use_embedded=off, quantization=Truncate, overflow=Wrap, mux_factor=0}
      mask prompts: input_bit_width "Input Bit Width"; coeff_bit_width "Coefficient Bit Width"; add_latency "Add Latency"; mult_latency "Mult Latency"; bram_latency "BRAM Latency"; use_hdl "Use behavioural HDL for multipliers"; use_embedded "Use embedded multipliers"; quantization "Quantization Behavior"; overflow "Overflow Behavior"; mux_factor "Multiplex factor (2^?)"
      mask help:
      | Used in FFT library. Used when result of
      | coeff*(a+jb)=b-ja
      mask StyleString: edit,edit,edit,edit,edit,checkbox,checkbox,popup(Truncate|Round  (unbiased: +/- Inf)|Round  (unbiased: Even Values)),popup(Wrap|Saturate|Error),edit
  twiddle_general_3mult : Subsystem  mask(twiddle_general_3mult_mux){Coeffs=getfield( getfield( get_param( gcb,'UserData' ), 'parameters'),'Coeffs'), StepPeriod=0, coeffs_bram=on, coeff_bit_width=18, input_bit_width=18, add_latency=3, mult_latency=4, bram_latency=4, arch=Virtex2Pro, use_hdl=off, use_embedded=off, quantization=Truncate, overflow=Wrap, mux_factor=0}
      mask prompts: Coeffs "Coefficients:"; StepPeriod "Coefficient Step Period (2^?)"; coeffs_bram "Store coefficients in BRAM"; coeff_bit_width "Coefficient Bit Width"; input_bit_width "Input Bit Width"; add_latency "Add Latency"; mult_latency "Mult Latency"; bram_latency "BRAM Latency"; arch "Architecture"; use_hdl "Use behavioral HDL for multlipliers"; use_embedded "Use embedded multipliers"; quantization "Quantization Behavior"; overflow "Overflow Behavior"; mux_factor "Multiplex factor (2^?)"
      mask help:
      | Used in biplex pipelined FFT. Takes advantage that
      | (a+bi)(c+di)=(c(a+b)-b(c+d))+i(b(c+d)+a(c-d)) to
      | save on multipliers at expense of adders.
      mask init:
      | twiddle_general_3mult_mux_init(gcb, ... 
      |     'Coeffs', Coeffs, ...
      |     'mux_factor', mux_factor, ...
      |     'StepPeriod', StepPeriod, ...
      |     'coeffs_bram', coeffs_bram, ...
      |     'coeff_bit_width', coeff_bit_width, ...
      |     'input_bit_width', input_bit_width, ...
      |     'add_latency', add_latency, ...
      |     'mult_latency', mult_latency, ...
      |     'bram_latency', bram_latency, ...
      |     'arch', arch, 'use_hdl', use_hdl, ...
      |     'use_embedded', use_embedded, ...
      |     'quantization', quantization, ...
      |     'overflow', overflow)
      settings: AttributesFormatString=|
      | arch=Virtex2Pro,
      |  input_bit_width=18,
      |  coeff_bit_width=18
      mask StyleString: edit,edit,checkbox,edit,edit,edit,edit,edit,popup(Virtex2Pro|Virtex5),checkbox,checkbox,popup(Truncate|Round  (unbiased: +/- Inf)|Round  (unbiased: Even Values)),popup(Wrap|Saturate|Error),edit
      mask CallbackString:
      | |||||||||use_hdl = get_param(gcb,'use_hdl');
      | visibs = get_param(gcb, 'MaskVisibilities');
      | if( strcmp(use_hdl,'on')),
      |     set_param(gcb, 'use_embedded','off');
      |     visibs{11} = 'off';
      | else,
      |     visibs{11} = 'on';
      | end
      | set_param(gcb, 'MaskVisibilities', visibs);
      | ||||
  twiddle_general_4mult : Subsystem  mask(twiddle_general_4mult_mux){Coeffs=0+0.29999999999999998889776975374843i, StepPeriod=0, coeffs_bram=on, coeff_bit_width=18, input_bit_width=18, add_latency=0, mult_latency=3, bram_latency=4, arch=Virtex2Pro, use_hdl=off, use_embedded=off, quantization=Round  (unbiased: Even Values), overflow=Wrap, mux_factor=0}
      mask prompts: Coeffs "Coefficients:"; StepPeriod "Coefficient Step Period (2^?)"; coeffs_bram "Store coefficients in BRAM"; coeff_bit_width "Coefficient Bit Width"; input_bit_width "Input Bit Width"; add_latency "Add Latency"; mult_latency "Mult Latency"; bram_latency "BRAM Latency"; arch "Architecture"; use_hdl "Use behavioural HDL for multipliers"; use_embedded "Use embedded multipliers"; quantization "Quantization Behavior"; overflow "Overflow Behavior"; mux_factor "Multiplex factor (2^?)"
      mask help:
      | Used in biplex pipelined FFT. Implements
      | (a+bi)(c+di) as (ac-bd)+i(ad+bc) with four
      | multipliers
      mask init:
      | twiddle_general_4mult_mux_init(gcb, ...
      |     'Coeffs', Coeffs, ...
      |     'mux_factor', mux_factor, ...
      |     'StepPeriod', StepPeriod, ...
      |     'coeffs_bram', coeffs_bram, ...
      |     'coeff_bit_width', coeff_bit_width, ...
      |     'input_bit_width', input_bit_width, ...
      |     'add_latency', add_latency, ...
      |     'mult_latency', mult_latency, ...
      |     'bram_latency', bram_latency, ...
      |     'arch', arch, ...
      |     'use_hdl', use_hdl, ...
      |     'use_embedded', use_embedded, ...
      |     'quantization', quantization, ...
      |     'overflow', overflow)
      settings: AttributesFormatString=|
      | arch=Virtex2Pro,
      |  input_bit_width=18,
      |  coeff_bit_width=18
      mask StyleString: edit,edit,checkbox,edit,edit,edit,edit,edit,popup(Virtex2Pro|Virtex5),checkbox,checkbox,popup(Truncate|Round  (unbiased: +/- Inf)|Round  (unbiased: Even Values)),popup(Wrap|Saturate|Error),edit
      mask CallbackString:
      | |||||||||use_hdl = get_param(gcb,'use_hdl');
      | visibs = get_param(gcb, 'MaskVisibilities');
      | if( strcmp(use_hdl,'on')),
      |     set_param(gcb, 'use_embedded','off');
      |     visibs{11} = 'off';
      | else,
      |     visibs{11} = 'on';
      | end
      | set_param(gcb, 'MaskVisibilities', visibs);||||
  twiddle_pass_through : Subsystem  mask(twiddle_pass_through){input_bit_width=18, coeff_bit_width=18, add_latency=3, mult_latency=4, bram_latency=4, use_hdl=off, use_embedded=off, quantization=Truncate, overflow=Wrap, mux_factor=0}
      mask prompts: input_bit_width "Input Bit Width"; coeff_bit_width "Coefficient Bit Width"; add_latency "Add Latency"; mult_latency "Mult Latency"; bram_latency "BRAM Latency"; use_hdl "Use behavioural HDL for multipliers"; use_embedded "Use embedded multipliers"; quantization "Quantization Behavior"; overflow "Overflow Behavior"; mux_factor "Multiplex factor (2^?)"
      mask help:
      | Used in FFT library. Used when coefficients
      | are 2^0 i.e just pass data through without delays
      mask StyleString: edit,edit,edit,edit,edit,checkbox,checkbox,popup(Truncate|Round  (unbiased: +/- Inf)|Round  (unbiased: Even Values)),popup(Wrap|Saturate|Error),edit
  twiddle_stage_2 : Subsystem  mask(twiddle_stage_2){FFTSize=5, input_bit_width=18, coeff_bit_width=18, add_latency=3, mult_latency=4, bram_latency=4, use_hdl=off, use_embedded=off, quantization=Truncate, overflow=Wrap, mux_factor=0}
      mask prompts: FFTSize "Size of FFT: (2^?)"; input_bit_width "Input Bit Width"; coeff_bit_width "Coefficient Bit Width"; add_latency "Add Latency"; mult_latency "Mult Latency"; bram_latency "BRAM Latency"; use_hdl "Use behavioural HDL for multipliers"; use_embedded "Use embedded multipliers"; quantization "Quantization Behavior"; overflow "Overflow Behavior"; mux_factor "Multiplex factor (2^?)"
      mask help:
      | Second stage in pipelined FFT. Takes
      | advantage of coefficients to be more efficient.
      mask StyleString: edit,edit,edit,edit,edit,edit,checkbox,checkbox,popup(Truncate|Round  (unbiased: +/- Inf)|Round  (unbiased: Even Values)),popup(Wrap|Saturate|Error),edit

== system ox_lib/biplex_core_mux ==
  pol1 : Inport  OutDataType=sfix(16)  OutScaling=2^0
  pol2 : Inport  Port=2  OutDataType=sfix(16)  OutScaling=2^0
  sync : Inport  Port=3  OutDataType=sfix(16)  OutScaling=2^0
  shift : Inport  Port=4  OutDataType=sfix(16)  OutScaling=2^0
  Constant : xbsIndex_r4/Constant  arith_type=Boolean  const=0  n_bits=1  bin_pt=1  explicit_period=off  period=1  equ=P=C  opselect=C  inp2=PCIN>>17  opr=+  inp1=P  carry=CIN  dbl_ovrd=off  block_type=constant
  fft_stage_n_mux : ox_lib/fft_stage_n_mux  SystemSampleTime=-1  FFTSize=4  FFTStage=1  input_bit_width=18  coeff_bit_width=18  delays_bram=off  coeffs_bram=off  MaxCoeffNum=16  quantization=Truncate  overflow=Wrap  add_latency=1  mult_latency=3  bram_latency=3  arch=Virtex2Pro  opt_target=Multipliers  use_hdl=on  use_embedded=off  dsp48_adders=off  mux_factor=4
      settings: AttributesFormatString=|
      | FFTSize=4, FFTStage=1,
      |  coeffs_bram=off,
      |  delays_bram=off
  fft_stage_n_mux1 : ox_lib/fft_stage_n_mux  SystemSampleTime=-1  FFTSize=4  FFTStage=1  input_bit_width=18  coeff_bit_width=18  delays_bram=off  coeffs_bram=off  MaxCoeffNum=16  quantization=Truncate  overflow=Wrap  add_latency=1  mult_latency=3  bram_latency=3  arch=Virtex2Pro  opt_target=Multipliers  use_hdl=on  use_embedded=off  dsp48_adders=off  mux_factor=4
      settings: AttributesFormatString=|
      | FFTSize=4, FFTStage=1,
      |  coeffs_bram=off,
      |  delays_bram=off
  fft_stage_n_mux2 : ox_lib/fft_stage_n_mux  SystemSampleTime=-1  FFTSize=4  FFTStage=1  input_bit_width=18  coeff_bit_width=18  delays_bram=off  coeffs_bram=off  MaxCoeffNum=16  quantization=Truncate  overflow=Wrap  add_latency=1  mult_latency=3  bram_latency=3  arch=Virtex2Pro  opt_target=Multipliers  use_hdl=on  use_embedded=off  dsp48_adders=off  mux_factor=4
      settings: AttributesFormatString=|
      | FFTSize=4, FFTStage=1,
      |  coeffs_bram=off,
      |  delays_bram=off
  out1 : Outport  OutDataType=sfix(16)  OutScaling=2^0
  out2 : Outport  Port=2  OutDataType=sfix(16)  OutScaling=2^0
  of : Outport  Port=3  OutDataType=sfix(16)  OutScaling=2^0
  sync_out : Outport  Port=4  OutDataType=sfix(16)  OutScaling=2^0
  wires:
  fft_stage_n_mux2/4 -> sync_out/1
  fft_stage_n_mux2/3 -> of/1
  fft_stage_n_mux2/2 -> out2/1
  fft_stage_n_mux2/1 -> out1/1
  sync/1 -> fft_stage_n_mux/4
  Constant/1 -> fft_stage_n_mux/3
  pol2/1 -> fft_stage_n_mux/2
  pol1/1 -> fft_stage_n_mux/1
  fft_stage_n_mux1/4 -> fft_stage_n_mux2/4
  fft_stage_n_mux1/3 -> fft_stage_n_mux2/3
  fft_stage_n_mux1/2 -> fft_stage_n_mux2/2
  fft_stage_n_mux1/1 -> fft_stage_n_mux2/1
  shift/1 -> fft_stage_n_mux/5, fft_stage_n_mux1/5, fft_stage_n_mux2/5
  fft_stage_n_mux/4 -> fft_stage_n_mux1/4
  fft_stage_n_mux/3 -> fft_stage_n_mux1/3
  fft_stage_n_mux/2 -> fft_stage_n_mux1/2
  fft_stage_n_mux/1 -> fft_stage_n_mux1/1
